simulink model "simulation1"  (Simulink 7.8)
settings: Solver=ode45  StartTime=0.0  StopTime=20  RelTol=1e-3
StopFcn:
  | plotQuadSimResult
values from neighbouring files (symbols this model uses):
  outerController = optimizer( con, obj, opt, [x2(:,1);ref2], u2(end:-1:1,1) )    [getOuterController.m]    (also in main.m = getOuterController(Ac, 'quadprog'))
  quad =     [quadData.mat]
  sys =     [quadData.mat]
  us = [0.700714285714 0.700714285714 0.700714285714 0.700714285714]    [quadData.mat]
libraries: simulink x1
settings Model: Creator=cjones  LastModifiedBy=milankorda

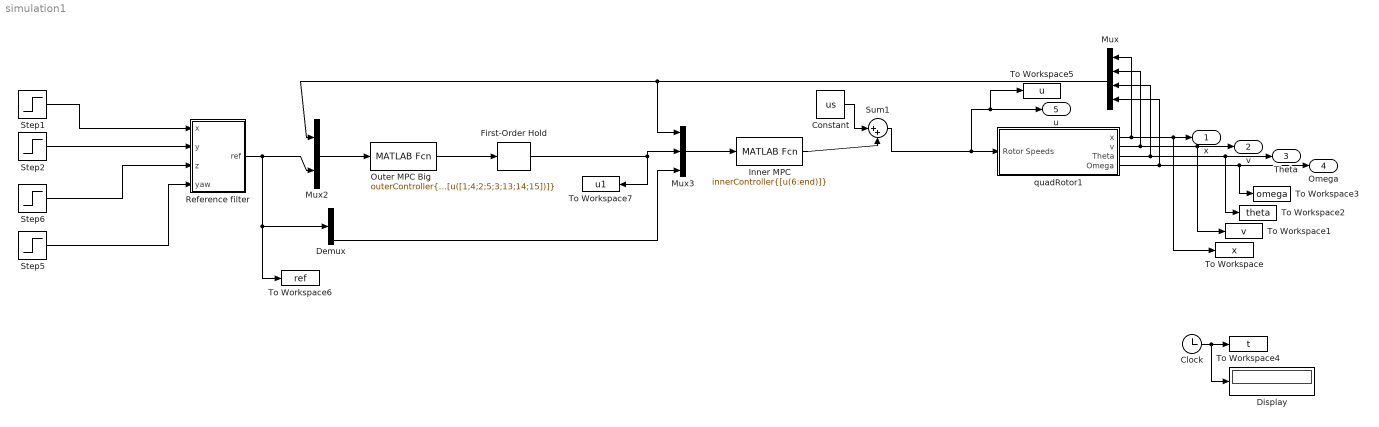
== system simulation1 ==
  Clock : Clock
  Constant : Constant  Value=us
  Demux : Demux
  Display : Display
  First-Order Hold : simulink/Discrete/First-Order Hold  DisableCoverage=on  Ts=quad.Ts2
  Inner MPC : MATLABFcn  MATLABFcn=innerController{[u(6:end)]}  OutputDimensions=4  OutputSignalType=real  SampleTime=sys.Ts
  Mux : Mux
  Mux2 : Mux  Inputs=[12 4]
  Mux3 : Mux  Inputs=[12 3 1]
  Outer MPC Big : MATLABFcn  MATLABFcn=outerController{[u([1;4;2;5;3;13;14;15])]}  OutputDimensions=3  OutputSignalType=real  SampleTime=quad.Ts2
  Reference filter : Subsystem
  Step1 : Step  After=3  SampleTime=0
  Step2 : Step  After=1.5  SampleTime=0
  Step5 : Step  After=pi  SampleTime=0
  Step6 : Step  After=2  SampleTime=0
  Sum1 : Sum  Inputs=|++
  To Workspace : ToWorkspace  VariableName=x  SampleTime=0.1  SaveFormat=Array
  To Workspace1 : ToWorkspace  VariableName=v  SampleTime=0.1  SaveFormat=Array
  To Workspace2 : ToWorkspace  VariableName=theta  SampleTime=0.1  SaveFormat=Array
  To Workspace3 : ToWorkspace  VariableName=omega  SampleTime=0.1  SaveFormat=Array
  To Workspace4 : ToWorkspace  VariableName=t  SampleTime=0.1  SaveFormat=Array
  To Workspace5 : ToWorkspace  VariableName=u  SampleTime=0.1  SaveFormat=Array
  To Workspace6 : ToWorkspace  VariableName=ref  SampleTime=0.1  SaveFormat=Array
  To Workspace7 : ToWorkspace  VariableName=u1  SampleTime=0.1  SaveFormat=Array
  quadRotor1 : Subsystem  mask{dist=off}
      mask prompts: dist "disturbance on/off"
  x : Outport
  v : Outport  Port=2
  Theta : Outport  Port=3
  Omega : Outport  Port=4
  u : Outport  Port=5
  wires:
  quadRotor1/1(x) -> x/1, To Workspace/1, Mux/1
  quadRotor1/2(v) -> v/1, To Workspace1/1, Mux/2
  quadRotor1/4(Omega) -> Omega/1, To Workspace3/1, Mux/4
  quadRotor1/3(Theta) -> Mux/3, Theta/1, To Workspace2/1
  Clock/1 -> To Workspace4/1, Display/1
  Mux/1 -> Mux2/1, Mux3/1
  Sum1/1 -> To Workspace5/1, u/1, quadRotor1/1(Rotor Speeds)
  Demux/4 -> Mux3/3
  Mux3/1 -> Inner MPC/1
  First-Order Hold/1 -> Mux3/2, To Workspace7/1
  Reference filter/1(ref) -> Mux2/2, Demux/1, To Workspace6/1
  Mux2/1 -> Outer MPC Big/1
  Outer MPC Big/1 -> First-Order Hold/1
  Constant/1 -> Sum1/1
  Inner MPC/1 -> Sum1/2
  Step1/1 -> Reference filter/1(x)
  Step6/1 -> Reference filter/3(z)
  Step5/1 -> Reference filter/4(yaw)
  Step2/1 -> Reference filter/2(y)

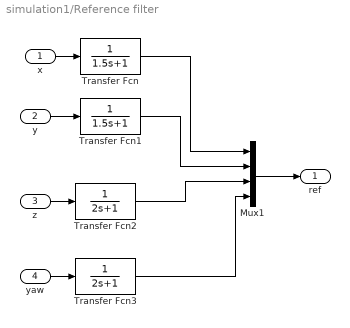
== system simulation1/Reference filter ==
  x : Inport
  y : Inport  Port=2
  z : Inport  Port=3
  yaw : Inport  Port=4
  Mux1 : Mux
  Transfer Fcn : TransferFcn  Denominator=[1.5 1]
  Transfer Fcn1 : TransferFcn  Denominator=[1.5 1]
  Transfer Fcn2 : TransferFcn  Denominator=[2 1]
  Transfer Fcn3 : TransferFcn  Denominator=[2 1]
  ref : Outport
  wires:
  x/1 -> Transfer Fcn/1
  y/1 -> Transfer Fcn1/1
  z/1 -> Transfer Fcn2/1
  yaw/1 -> Transfer Fcn3/1
  Mux1/1 -> ref/1
  Transfer Fcn/1 -> Mux1/1
  Transfer Fcn1/1 -> Mux1/2
  Transfer Fcn2/1 -> Mux1/3
  Transfer Fcn3/1 -> Mux1/4

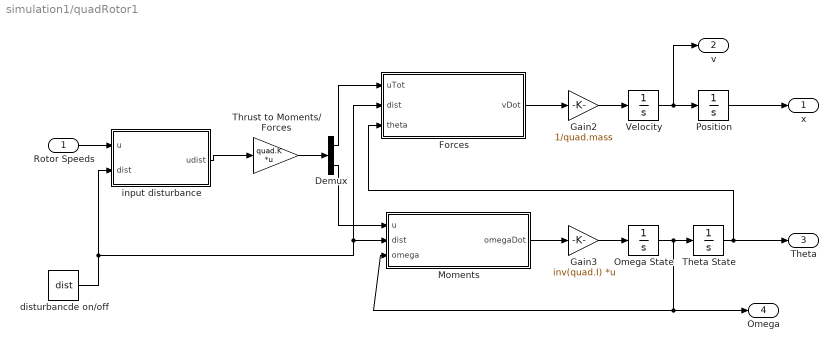
== system simulation1/quadRotor1 ==
  Rotor Speeds : Inport
  Demux : Demux  Outputs=[1 3]
  Forces : MATLAB Function  TreatAsAtomicUnit=on
  Gain2 : Gain  Gain=1/quad.mass
  Gain3 : Gain  Gain=inv(quad.I)  Multiplication=Matrix(K*u)
  Moments : MATLAB Function  TreatAsAtomicUnit=on
  Omega State : Integrator  InitialCondition=[0;0;0]
  Position : Integrator  InitialCondition=[0;0;0]
  Theta State : Integrator  InitialCondition=[0;0;0]
  Thrust to Moments/ Forces : Gain  Gain=quad.K  Multiplication=Matrix(K*u)
  Velocity : Integrator  InitialCondition=[0;0;0]
  disturbancde on/off : Constant  Value=dist
  input disturbance : MATLAB Function  TreatAsAtomicUnit=on
  x : Outport
  v : Outport  Port=2
  Theta : Outport  Port=3
  Omega : Outport  Port=4
  wires:
  Thrust to Moments/ Forces/1 -> Demux/1
  Gain3/1 -> Omega State/1
  Theta State/1 -> Theta/1, Forces/3(theta)
  Demux/1 -> Forces/1(uTot)
  Velocity/1 -> Position/1, v/1
  Rotor Speeds/1 -> input disturbance/1(u)
  Position/1 -> x/1
  Omega State/1 -> Theta State/1, Omega/1, Moments/3(omega)
  Moments/1(omegaDot) -> Gain3/1
  Demux/2 -> Moments/1(u)
  Forces/1(vDot) -> Gain2/1
  Gain2/1 -> Velocity/1
  input disturbance/1(udist) -> Thrust to Moments/ Forces/1
  disturbancde on/off/1 -> input disturbance/2(dist), Forces/2(dist), Moments/2(dist)

== matlab function quadRotor1/Forces ==
  data: uTot input double; dist input double; vDot output double; theta input double; quad parameter double
function vDot = forces(uTot,dist, theta, quad)
%#codegen

% Rotation from body to interial frame 
roll = theta(1); pitch = theta(2); yaw = theta(3);
R = [1 0 0;0 cos(roll) -sin(roll);0 sin(roll) cos(roll)];
R = R*[cos(pitch) 0 sin(pitch); 0 1 0; -sin(pitch) 0 cos(pitch)];
R = R*[cos(yaw) -sin(yaw) 0; sin(yaw) cos(yaw) 0; 0 0 1];

% Forces
g = 9.81;
if(dist)
    d = -quad.mass*(1)*[0;0;1]; %gravity error
else
    d = [0;0;0];
end
vDot = -quad.mass*(g)*[0;0;1] + uTot*R*[0;0;1] + d;

== matlab function quadRotor1/Moments ==
  data: u input double; dist input double; omega input double; quad parameter double; omegaDot output double
function omegaDot = moments(u, dist, omega, quad)
%#codegen
if(dist)
    d = [1;1;1] + +[0;0;40]*(rand(1)-0.5) + 4*(rand(3,1)-0.5); %disturbance 
else
    d = [0;0;0];
end
% Rotational derivative
omegaDot = -cross(omega, quad.I*omega) + u + d ;

== matlab function quadRotor1/input disturbance ==
  data: u input double; udist output double; dist input double
function udist = inputDist(u,dist)
%#codegen
if(dist)
    udist = u + 1*[-0.05;0.02;0.03;-0.01];
else
    udist = u;
end
